simulink model "ENERGYMANAGEMENT0x2E"  (R2023b)
settings: Solver=VariableStepAuto  StartTime=0.0  StopTime=10  RelTol=1e-3  EnableMultiTasking=on
PreLoadFcn:
  |  SurfaceMountedPMSMFieldOrientedControlData
values from neighbouring files (symbols this model uses):
  F = 0.005    [SurfaceMountedPMSMFieldOrientedControlData.m]
  Fsw = 8000    [SurfaceMountedPMSMFieldOrientedControlData.m]
  Ts = 20e-6    (= 2e-05)    [SurfaceMountedPMSMFieldOrientedControlData.m]
undefined symbols (not defined in the file or in its folder): DiscIntNeverNeededParam, gcbh, Ion, Lithium, sps_rtmsupport
libraries: simulink x16, spsDiodeLib x6, spsSeriesRLCBranchLib x4, slpidlib x3, spsCurrentMeasurementLib x2, simulink_extras x2, spsMeanLib x2, spsSecondOrderFilterLib x2, spsIdealSwitchLib x2, spsPermanentMagnetSynchronousMachineLib x1, spsBatteryLib x1, spsMosfetLib x1
(part 1 of 2)
settings Model: SimulationMode=accelerator  Creator=The MathWorks, Inc.  LastModifiedBy=osman
settings SolverCC: AlgebraicLoopSolver=TrustRegion
settings DataIOCC: SaveOutput=off  SignalLogging=off  DSMLogging=off  SaveTime=off  ReturnWorkspaceOutputs=off
settings DebuggingCC: UnconnectedInputMsg=warning  UnconnectedOutputMsg=warning  UnconnectedLineMsg=warning
settings ModelReferenceCC: EnableRefExpFcnMdlSchedulingChecks=on
settings RTWCC: DLArmComputeVersion=19.05

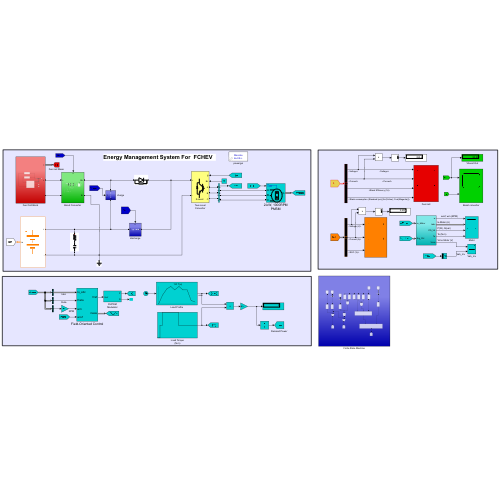
[thumbnail: Simulink's stored preview of the top-level diagram]
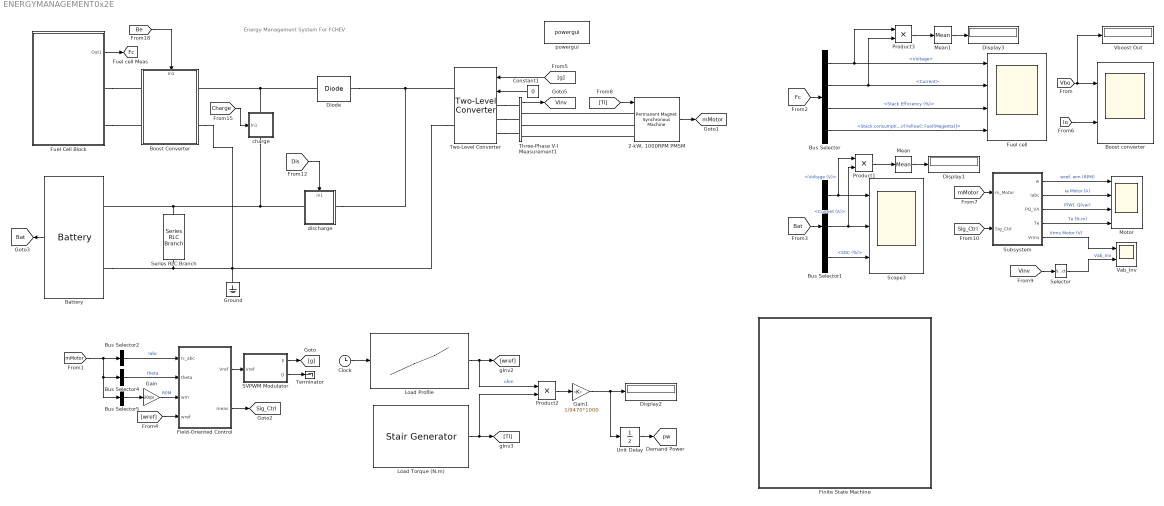
== system ENERGYMANAGEMENT0x2E ==
  note: Energy Management System For FCHEV
  "2-kW, 1000RPM PMSM" : spsPermanentMagnetSynchronousMachineLib/Permanent Magnet Synchronous Machine  NbPhases=3  FluxDistribution=Sinusoidal  RotorType=Round  MechanicalLoad=Torque Tm  PresetModel=No  ShowDetailedParameters=on  MeasurementBus=off  Resistance=0.01  Inductance=8.5e-3  dqInductances=[8.5e-3,8.5e-3]  La=0.002  MachineConstant=Flux linkage established by magnets (V.s)  Flux=0.175  VoltageCst=95.2245  TorqueCst=0.7875  Flat=120  Mechanical=[0.03 ,F 3]  PolePairs=2  InitialConditions=[0,0, 0,0]  InitialConditions5ph=[0 0 0 0 0 0]  RefAngle=90 degrees behind phase A axis (modified Park)  IterativeDiscreteModel=Trapezoidal robust  TsBlock=2e-5  TsPowergui=0
  Battery : spsBatteryLib/Battery  BatType=Lithium-Ion  ShowTempParam=off  ThermalPreset=no  ShowAgeParam=off  NomV=88  NomQ=11  SOC=75  Batt_Tr=30  PresetModel=on  MaxQ=11  MinV=66  FullV=102.4309  Dis_rate=4.7826  R=0.08  Normal_OP=9.9478  expZone="[95.074     0.540435]"  current=[6.5 13 32.5]  Units=Time  Tci=20  NomT=20  T2=-30  MaxQ2=4.8  FullV2=7.1  Normal_OP2=5.655  expZone2="[6.58           1]"  Rca=0.6  ti=2000  Dp=0  Neq0=0  Tsim=1e6  Ta1=25  Qeol=5.4*0.9  Reol=0.013333*1.2  Char_age=[2.3478, 3]  Dis_age=[2.3478, 10]  N1=1500  N2=10500  N3=1000  N4=1400  Ta2=45  N5=950
  Boost Converter : Subsystem
      settings: PortSchema="{\"entries\":[{\"content\":{\"sides\":[{\"content\":{\"connectorIds\":[\"LConn1\",\"LConn2\"]},\"type\":\"ConnectorPlacement.EquallySpacedRectSide\",\"uuid\":\"724820d7-5254-4590-9883-e42ece5a36b7\"},{\"content\":{\"connectorIds\":[\"RConn1\",\"RConn2\"],\"side\":\"RIGHT\"},\"type\":\"ConnectorPlacement.EquallySpacedRectSide\",\"uuid\":\"efd78358-38e4-437c-85ef-e8b0a8150418\"},{\"content\":{\"connectorIds\":[\"In1\"],\"side\":\"TOP\"},\"type\":\"ConnectorPlacement.EquallySpacedRectSide\",\"uuid\":\"51cbfe1b-7a5a-4465-8e4f-b2b0baad5ef4\"}]},\"type\":\"ConnectorPlacement.EquallySpacedConnector\",\"uuid\":\"bbc907d0-d787-42dc-8369-3440b3d38849\"}],\"packageUris\":[\"http://schema.mathworks.com/mf0/Connector/R2020b\"],\"version\":\"1.0\"}"
  Boost converter : Scope  NumInputPorts=2
  Bus Selector : BusSelector  OutputSignals=Voltage,Current,Stack Efficiency (%),Stack consumption (Standard lpm) [Air(Yellow); Fuel(Magenta)]
  Bus Selector1 : BusSelector  OutputSignals=Voltage (V),Current (A),SOC (%)
  Bus Selector2 : BusSelector  OutputSignals=Stator current is_a (A),Stator current is_b (A),Stator current is_c (A)  OutputAsBus=on
  Bus Selector4 : BusSelector  OutputSignals=Rotor angle thetam (rad)  OutputAsBus=on
  Bus Selector5 : BusSelector  OutputSignals=Rotor speed wm (rad/s)  OutputAsBus=on
  Clock : Clock
  Constant1 : Constant  Value=0
  Diode : spsDiodeLib/Diode  Ron=0.001  Lon=0  Vf=0.8  IC=0  UseSnubber=0  Rs=1e5  Cs=250e-9  Measurements=off
  Display1 : Display
  Display2 : Display
  Display3 : Display
  Field-Oriented Control : Subsystem  DialogController=POWERSYS.PowerSysDialog  LoadFcn=sps_rtmsupport('LoadFcn',gcbh);  StartFcn=sps_rtmsupport('StartFcn',gcbh);  StopFcn=sps_rtmsupport('StopFcn',gcbh);  mask(Field-Oriented Controller (FOC) of a PMSM drive){Kp_wreg=0.25, Ki_wreg=25, Limit_wreg=35, Kp_Ireg=0.2, Ki_Ireg=10, Limits_Ireg=2, p=3, Ts=2e-5}
      mask prompts: Kp_wreg "Proportional gain"; Ki_wreg "Integral gain"; Limit_wreg "Output (current) limit"; Kp_Ireg "Proportional gain"; Ki_Ireg "Integral gain"; Limits_Ireg "Output limit"; p "Number of pole pairs:"; Ts "Sample time (s)"
      settings: AttributesFormatString=\n  CopyFcn=sps_rtmsupport('CopyFcn',gcbh); powericon('psbloadfunction',gcbh,'gotofrom','UpdateGotoTag');  DeleteFcn=sps_rtmsupport('DeleteFcn',gcbh);  UndoDeleteFcn=sps_rtmsupport('UndoDeleteFcn',gcbh);  ModelCloseFcn=sps_rtmsupport('ModelCloseFcn',gcbh);  PreSaveFcn=sps_rtmsupport('PreSaveFcn',gcbh);  PostSaveFcn=sps_rtmsupport('PostSaveFcn',gcbh);  NameChangeFcn=sps_rtmsupport('NameChangeFcn',gcbh);  PreCopyFcn=sps_rtmsupport('PreCopyFcn',gcbh);  OpenFcn=sps_rtmsupport('OpenFcn',gcbh, [-1 2 -3 4 5 6 7 17 22 23]);  CloseFcn=sps_rtmsupport('CloseFcn',gcbh);  PreDeleteFcn=sps_rtmsupport('PreDeleteFcn',gcbh);
      mask Help: helpview(psbhelp);
      mask DialogControl Container11 Prompt: Control parameters
      mask DialogControl Container12 Prompt: Speed regulator
      mask DialogControl Container8 Prompt: Current regulators
  Finite State Machine : Subsystem
  Fuel Cell Block : Subsystem
  Fuel cell : Scope  NumInputPorts=4
  Gain : Gain  Gain=30/pi
  Gain1 : Gain  Gain=1/9470*1000
  Ground : spsGroundLib/Ground  LConnTagsString=a
  Load Profile : Lookup_n-D  NumberOfTableDimensions=1  BreakpointsForDimension1=[0 1 2 3 4 5 6 7 8 9 ]  BreakpointsForDimension2=[0 571.55 685.8 800.15 914.4 1028.8 1143.1 1257.4 1371.7 1486 1600.3 1714.6 1828.9 1943.2 2057.5 2171.8 2286.1 2400.5 2514.7 2629.1 2743.3 2857.7 2971.9 3086.3 3200.5 3314.9 3429.2]  Table=[0 500 850 1000 800 1000 800 800 200 100 ]  InternalRulePriority=Speed  RndMeth=Simplest
  Load Torque (N.m) : spsStairGeneratorLib/Stair Generator  t=[0 0.5 1 1.5 5 9]  e=[5 , 5 10 15 10 10 ]  Ts=Ts
  Mean : spsMeanLib/Mean  Freq=60  Vinit=0  Ts=2e-5
  Mean1 : spsMeanLib/Mean  Freq=60  Vinit=0  Ts=2e-5
  Motor : Scope  NumInputPorts=4
  Product1 : Product
  Product2 : Product
  Product3 : Product
  SVPWM Modulator : Subsystem  DialogController=POWERSYS.PowerSysDialog  LoadFcn=sps_rtmsupport('LoadFcn', gcbh);  StartFcn=sps_rtmsupport('StartFcn', gcbh);  StopFcn=sps_rtmsupport('StopFcn', gcbh);  mask(Unified PWM Modulator for a 2-level, 3-phase converter){PWMmethod=Space Vector PWM (SVPWM) with pulse averaging, Fsw=Fsw, Ts=Ts}
      mask prompts: PWMmethod "PWM method"; Fsw "Switching frequency (Hz):"; Ts "Sample time (s):"
      mask help:
      | Generate pulses for PWM-controlled two-level, three-phase power electronics converter with pulse averaging capability.
      |
      | The pulses generation can be perform using one of the following Pulse-Width Modulation (PWM) methods:
      | 1. Sinusoidal PWM (SPWM)
      | 2. Sinusoidal PWM (SPWM) with pulse averaging
      | 3. Space Vector PWM (SVPWM)
      | 4. Space Vector PWM (SVPWM) with pulse averaging
      | 5. 30 degrees discontinuous PWM
      |
      | When a PWM method with pulse averaging is selected, the output pulses are averaged over one sample time. (Pulses value will range from 0 to 1)
      mask init:
      | switch PWMmethod
      |     case 1 % SPWM
      |         ZeroOrderHold_Ts=-1;
      |         Pavg=0;
      |     case 2 % SPWM with pulse averaging
      |         ZeroOrderHold_Ts=-1;
      |         Pavg=1;
      |     case 3  % SVPWM
      |         ZeroOrderHold_Ts=-1;
      |         Pavg=0;
      |     case 4  % SVPWM with pulse averaging
      |         ZeroOrderHold_Ts=-1;
      |         Pavg=1;
      |     case 5  % 30 degrees discontinuous PWM
      |         ZeroOrderHold_Ts=1/Fsw/2;
      |         Pavg=0;
      | end
      settings: CopyFcn=sps_rtmsupport('CopyFcn', gcbh);  DeleteFcn=sps_rtmsupport('DeleteFcn', gcbh);  UndoDeleteFcn=sps_rtmsupport('UndoDeleteFcn', gcbh);  ModelCloseFcn=sps_rtmsupport('ModelCloseFcn', gcbh);  PreSaveFcn=sps_rtmsupport('PreSaveFcn', gcbh);  PostSaveFcn=sps_rtmsupport('PostSaveFcn', gcbh);  NameChangeFcn=sps_rtmsupport('NameChangeFcn', gcbh);  PreCopyFcn=sps_rtmsupport('PreCopyFcn', gcbh);  OpenFcn=sps_rtmsupport('OpenFcn', gcbh, [1]);  CloseFcn=sps_rtmsupport('CloseFcn', gcbh);  PreDeleteFcn=sps_rtmsupport('PreDeleteFcn', gcbh);
      mask TypeOptions PWMmethod: Sinusoidal PWM (SPWM) | Sinusoidal PWM (SPWM) wirh pulse averaging | Space Vector PWM (SVPWM) | Space Vector PWM (SVPWM) with pulse averaging | 30 degrees discontinuous PWM
  Scope3 : Scope  NumInputPorts=3
  Selector : Selector  InputPortWidth=3  IndexOptions=Index vector (dialog)  Indices=1  OutputSizes=1
  Series RLC Branch : spsSeriesRLCBranchLib/Series RLC Branch  LConnTagsString=__new0  RConnTagsString=__new0  BranchType=RC  Resistance=1  Inductance=1e-3  SetiL0=off  InitialCurrent=0  Capacitance=1e-4  Setx0=on  InitialVoltage=92  Measurements=None
  Subsystem : Subsystem
  Terminator : Terminator
  Three-Phase V-I Measurement1 : spsThreePhaseVIMeasurementLib/Three-Phase V-I Measurement  VoltageMeasurement=phase-to-phase  SetLabelV=off  LabelV=Vabc  Vpu=off  VpuLL=off  CurrentMeasurement=no  SetLabelI=off  LabelI=Iabc  Ipu=off  Pbase=100e6  Vbase=500e3  OutputType=Complex  PhasorSimulation=off  PSBequivalent=0
  Two-Level Converter : spsTwoLevelConverterLib/Two-Level Converter  ModelType=Switching function  Ron=1e-3  Rs=1e6  Cs=inf  Vforward=[0,0]  Ron_Diode=1e-3  Rs_Diode=1e6  Cs_Diode=inf  Vf_Diode=0  Rs_CurrentSource=inf  Ron_ACsource=1e-3
  Unit Delay : UnitDelay  SampleTime=2e-5  HasFrameUpgradeWarning=on
  Vab_Inv : Scope  NumInputPorts=2
  Vboost Out : Display
  charge : Subsystem
      settings: PortSchema="{\"entries\":[{\"content\":{\"sides\":[{\"content\":{\"connectorIds\":[\"LConn1\"]},\"type\":\"ConnectorPlacement.EquallySpacedRectSide\",\"uuid\":\"542812f3-0075-41f7-b004-faadc5b4cb6c\"},{\"content\":{\"connectorIds\":[\"RConn1\"],\"side\":\"RIGHT\"},\"type\":\"ConnectorPlacement.EquallySpacedRectSide\",\"uuid\":\"a1adf09c-e9ea-4226-86a1-520823d20346\"},{\"content\":{\"connectorIds\":[\"In1\"],\"side\":\"TOP\"},\"type\":\"ConnectorPlacement.EquallySpacedRectSide\",\"uuid\":\"e7c1831b-3d2b-475c-93da-3ac83c790107\"}]},\"type\":\"ConnectorPlacement.EquallySpacedConnector\",\"uuid\":\"19c42b2a-b3c4-4efa-a5c9-bfe092eb0a4e\"}],\"packageUris\":[\"http://schema.mathworks.com/mf0/Connector/R2020b\"],\"version\":\"1.0\"}"
  discharge : Subsystem
      settings: PortSchema="{\"entries\":[{\"content\":{\"sides\":[{\"content\":{\"connectorIds\":[\"LConn1\"]},\"type\":\"ConnectorPlacement.EquallySpacedRectSide\",\"uuid\":\"542812f3-0075-41f7-b004-faadc5b4cb6c\"},{\"content\":{\"connectorIds\":[\"RConn1\"],\"side\":\"RIGHT\"},\"type\":\"ConnectorPlacement.EquallySpacedRectSide\",\"uuid\":\"a1adf09c-e9ea-4226-86a1-520823d20346\"},{\"content\":{\"connectorIds\":[\"In1\"],\"side\":\"TOP\"},\"type\":\"ConnectorPlacement.EquallySpacedRectSide\",\"uuid\":\"e7c1831b-3d2b-475c-93da-3ac83c790107\"}]},\"type\":\"ConnectorPlacement.EquallySpacedConnector\",\"uuid\":\"19c42b2a-b3c4-4efa-a5c9-bfe092eb0a4e\"}],\"packageUris\":[\"http://schema.mathworks.com/mf0/Connector/R2020b\"],\"version\":\"1.0\"}"
  powergui : spspowerguiLib/powergui  Priority=1  SimulationMode=Discrete  SampleTime=Ts  frequency=60  Iterations=50  frequencyindice=0  Pbase=100e6  ErrMax=1e-4  UnitsV=kV  UnitsW=MW  buscounter=0  FunctionMessages=off  echomessages=off  EnableUseOfTLC=off  CurrentSourceSwitches=off  DisableSnubberDevices=off  DisableRonSwitches=off  DisableVfSwitches=off  DisplayEquations=off  AutomaticDiscreteSolvers=off  SolverType=Tustin/Backward Euler (TBE)  Interpol=off  ExternalGateDelay=off  methode=off  Ts=100  x0status=blocks  SPID=on  SwTol=0  HookPort=off  NonlinearTolerance=1e-4  nMaxIteration=100  ContinueOnMaxIteration=off  RestoreLinks=warning  ResistiveCurrentMeasurement=off  Frange=[0:2:500]  Ylog=off  Xlog=on  ShowGrid=off  save=off  variable=ZData  structure=Scope_Compare  ZoomFFT=off  StartTime=0.75  cycles=1  DisplayStyle=1  fundamental=100  FreqAxis=off  MaxFrequency=25000  frequencyindicesteady=1  RmsSteady=1  display=off
  tag scope: Bat=global, Fc=global, Sig_Ctrl=global, Vinv=global, mMotor=global, pw=global
  wires:
  Field-Oriented Control/1(Vref) -> SVPWM Modulator/1(Vref)
  Field-Oriented Control/2(meas) -> [Sig_Ctrl]
  [wref] -> Field-Oriented Control/4(wref)
  [mMotor] -> Bus Selector2/1, Bus Selector4/1, Bus Selector5/1
  Bus Selector2/1 -> Field-Oriented Control/1(Is_abc)  "Iabc"
  "2-kW, 1000RPM PMSM"/1 -> [mMotor]
  Constant1/1 -> Two-Level Converter/2
  Three-Phase V-I Measurement1/1 -> [Vinv]
  [g] -> Two-Level Converter/1
  Bus Selector5/1 -> Gain/1
  Gain/1 -> Field-Oriented Control/3(wm)  "RPM"
  Bus Selector4/1 -> Field-Oriented Control/2(theta)  "theta"
  SVPWM Modulator/1(P) -> [g]
  SVPWM Modulator/2(D) -> Terminator/1
  Battery/1 -> [Bat]
  Load Torque (N.m)/1 -> Product2/2, [Tl]
  Clock/1 -> Load Profile/1
  Load Profile/1 -> Product2/1, [wref]  "ohm"
  [Tl] -> "2-kW, 1000RPM PMSM"/1
  [Sig_Ctrl] -> Subsystem/2(Sig_Ctrl)
  Subsystem/3(PQ_VA) -> Motor/3  "P(W), Q(var)"
  [Vinv] -> Selector/1
  Subsystem/5(Vrms) -> Vab_Inv/1  "Vrms Motor (V)"
  Subsystem/4(Te) -> Motor/4  "Te (N.m)"
  [Bat] -> Bus Selector1/1
  Subsystem/2(Iabc) -> Motor/2  "Ia Motor (A)"
  [Vbo] -> Vboost Out/1, Boost converter/1
  Subsystem/1(w) -> Motor/1  "wref, wm (RPM)"
  Bus Selector/4 -> Fuel cell/4  "<Stack consumption (Standard lpm) [Air(Yellow); Fuel(Magenta)]>"
  Bus Selector/2 -> Product3/2, Fuel cell/2  "<Current>"
  [mMotor] -> Subsystem/1(m_Motor)
  [Fc] -> Bus Selector/1
  Bus Selector/3 -> Fuel cell/3  "<Stack Efficiency (%)>"
  Bus Selector/1 -> Product3/1, Fuel cell/1  "<Voltage>"
  [Io] -> Boost converter/2
  Selector/1 -> Vab_Inv/2  "Vab_Inv"
  Bus Selector1/1 -> Product1/1, Scope3/1  "<Voltage (V)>"
  Bus Selector1/2 -> Product1/2, Scope3/2  "<Current (A)>"
  Bus Selector1/3 -> Scope3/3  "<SOC (%)>"
  Fuel Cell Block/1(Out1) -> [Fc]
  Product2/1 -> Gain1/1
  Gain1/1 -> Unit Delay/1, Display2/1
  Unit Delay/1 -> [pw]
  [Dis] -> discharge/1(In1)
  [Charge] -> charge/1(In1)
  [Be] -> Boost Converter/1(In1)
  Product1/1 -> Mean/1
  Mean/1 -> Display1/1
  Mean1/1 -> Display3/1
  Product3/1 -> Mean1/1
  connections:
  "2-kW, 1000RPM PMSM"/LConn1 -- Three-Phase V-I Measurement1/RConn1
  Two-Level Converter/LConn3 -- Three-Phase V-I Measurement1/LConn3
  "2-kW, 1000RPM PMSM"/LConn2 -- Three-Phase V-I Measurement1/RConn2
  Two-Level Converter/LConn1 -- Three-Phase V-I Measurement1/LConn1
  Two-Level Converter/LConn2 -- Three-Phase V-I Measurement1/LConn2
  "2-kW, 1000RPM PMSM"/LConn3 -- Three-Phase V-I Measurement1/RConn3
  Fuel Cell Block/RConn2 -- Boost Converter/LConn2
  Fuel Cell Block/RConn1 -- Boost Converter/LConn1
  Two-Level Converter/RConn2 -- Series RLC Branch/RConn1 -- Battery/LConn2 -- Ground/LConn1 -- Boost Converter/RConn2
  discharge/LConn1 -- charge/RConn1 -- Series RLC Branch/LConn1 -- Battery/LConn1
  Diode/RConn1 -- discharge/RConn1 -- Two-Level Converter/RConn1
  Diode/LConn1 -- charge/LConn1 -- Boost Converter/RConn1

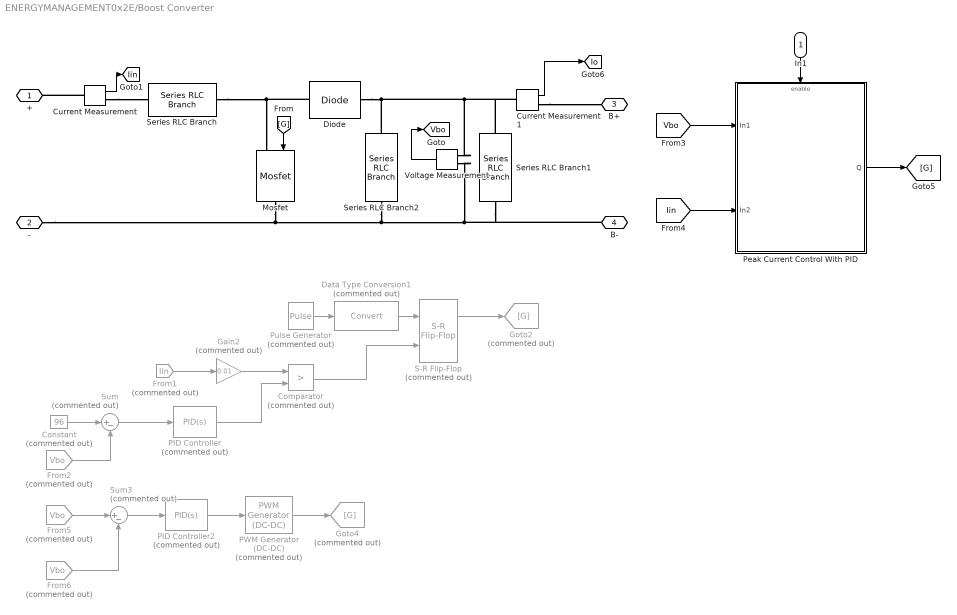
== system ENERGYMANAGEMENT0x2E/Boost Converter ==
  In1 : Inport
  Comparator : RelationalOperator  Commented=on  Operator=>  OutDataTypeStr=boolean  RndMeth=Simplest  InputSameDT=off
  Constant : Constant  Commented=on  Value=96
  Current Measurement : spsCurrentMeasurementLib/Current Measurement  PhasorSimulation=off  OutputType=Complex  PSBequivalent=0
  Current Measurement1 : spsCurrentMeasurementLib/Current Measurement  PhasorSimulation=off  OutputType=Complex  PSBequivalent=0
  Data Type Conversion1 : DataTypeConversion  Commented=on  SaturateOnIntegerOverflow=off  RndMeth=Floor
  Diode : spsDiodeLib/Diode  Ron=0.001  Lon=0  Vf=0  IC=0  UseSnubber=0  Rs=5e3  Cs=250e-9  Measurements=off
  From1 : From  Commented=on  GotoTag=Iin  TagVisibility=global
  From2 : From  Commented=on  GotoTag=Vbo  TagVisibility=global
  From5 : From  Commented=on  GotoTag=Vbo  TagVisibility=global
  From6 : From  Commented=on  GotoTag=Vbo  TagVisibility=global
  Gain2 : Gain  Commented=on  Gain=0.01
  Goto2 : Goto  Commented=on  GotoTag=G
  Goto4 : Goto  Commented=on  GotoTag=G
  Mosfet : spsMosfetLib/Mosfet  Ron=0.05  Lon=0  Rd=0.01  Vfd=0  IC=0  Rs=1e5  Cs=inf  Measurements=off
  PID Controller : slpidlib/PID Controller  Commented=on  Controller=PID  Form=Parallel  TimeDomain=Continuous-time  UseExternalTs=off  SampleTime=-1  IntegratorMethod=Forward Euler  FilterMethod=Forward Euler  ControllerParametersSource=internal  P=0.01  I=0.1  UseKiTs=off  D=0.001  N=100  UseFilter=on  TunerSelectOption=Transfer Function Based (PID Tuner App)  InitialConditionSource=internal  InitialConditionForIntegrator=0  InitialConditionForFilter=0  DifferentiatorICPrevScaledInput=0  ExternalReset=none  TrackingMode=off  Kt=1  LimitOutput=on  SatLimitsSource=internal  UpperSaturationLimit=0.80  LowerSaturationLimit=0  LinearizeAsGain=on  AntiWindupMode=none  Kb=1  LimitIntegrator=off  UpperIntegratorSaturationLimit=inf  LowerIntegratorSaturationLimit=-inf  POutMin=[]  POutMax=[]  IOutMin=[]  IOutMax=[]  DOutMin=[]  DOutMax=[]  NOutMin=[]  NOutMax=[]  SumOutMin=[]  SumOutMax=[]  SaturationOutMin=[]  SaturationOutMax=[]  PParamMin=[]  PParamMax=[]  IParamMin=[]  IParamMax=[]  DParamMin=[]  DParamMax=[]  NParamMin=[]  NParamMax=[]  KbParamMin=[]  KbParamMax=[]  KtParamMin=[]  KtParamMax=[]  KbOutMin=[]  KbOutMax=[]  KtOutMin=[]  KtOutMax=[]  IntegratorOutMin=[]  IntegratorOutMax=[]  FilterOutMin=[]  FilterOutMax=[]  SumI1OutMin=[]  SumI1OutMax=[]  SumI2OutMin=[]  SumI2OutMax=[]  SumI3OutMin=[]  SumI3OutMax=[]  SumI4OutMin=[]  SumI4OutMax=[]  SumDOutMin=[]  SumDOutMax=[]  DifferentiatorOutMin=[]  DifferentiatorOutMax=[]  FilterDiffOutCoefMin=[]  FilterDiffOutCoefMax=[]  ReciprocalOutMin=[]  ReciprocalOutMax=[]  SumDenOutMin=[]  SumDenOutMax=[]  SumNumOutMin=[]  SumNumOutMax=[]  DivideOutMin=[]  DivideOutMax=[]  UdiffTsProdOutMin=[]  UdiffTsProdOutMax=[]  NTsProdOutMin=[]  NTsProdOutMax=[]  UintegralTsProdOutMin=[]  UintegralTsProdOutMax=[]  UngainTsProdOutMin=[]  UngainTsProdOutMax=[]  ClampingZeroOutDataTypeStr=Inherit: Inherit via back propagation  ClampingZeroOutMin=[]  ClampingZeroOutMax=[]  FilterDenConstantOutDataTypeStr=Inherit: Inherit via back propagation  FilterDenConstantOutMin=[]  FilterDenConstantOutMax=[]  PCopyOutDataTypeStr=Inherit: Inherit via back propagation  PCopyOutMin=[]  PCopyOutMax=[]  NCopyOutDataTypeStr=Inherit: Inherit via back propagation  NCopyOutMin=[]  NCopyOutMax=[]  IntegratorContinuousStateAttributes=''  IntegratorStateMustResolveToSignalObject=off  IntegratorRTWStateStorageClass=Auto  FilterContinuousStateAttributes=''  FilterStateMustResolveToSignalObject=off  FilterRTWStateStorageClass=Auto  ParallelPVariant=InternalParameters  IdealPVariant=Disabled  IVariant=InternalParameters  DVariant=InternalParameters  IntegratorVariant=Continuous  SatVariant=Enabled  AWVariant=Passthrough  PCopyVariant=Disabled  TRVariant=Disabled  FdbkBlocksVariant=Forward  IdealPFdbkVariant=Disabled  SatFdbkVariant=Disabled  DerivativeFilterVariant=ContFilter  NVariant=InternalParameters  NCopyVariant=Disabled  FilterICVariant=InternalICsFilter  IntegratorICVariant=InternalICs  ExternalResetVariant=Disabled  TRSumVariant=Passthrough  SumFdbkVariant=Disabled  SumVariant=Sum_PID  TsampFilterVariant=InternalTs  TsampNgainVariant=Passthrough  TsampIntegralVariant=Disabled_SignalSpec  ExternalSaturationOutDataTypeStr=Inherit: Same as second input
  PID Controller2 : slpidlib/PID Controller  Commented=on  Controller=PID  Form=Parallel  TimeDomain=Continuous-time  UseExternalTs=off  SampleTime=-1  IntegratorMethod=Forward Euler  FilterMethod=Forward Euler  ControllerParametersSource=internal  P=0.01  I=0.1  UseKiTs=off  D=0.001  N=100  UseFilter=on  TunerSelectOption=Transfer Function Based (PID Tuner App)  InitialConditionSource=internal  InitialConditionForIntegrator=0  InitialConditionForFilter=0  DifferentiatorICPrevScaledInput=0  ExternalReset=none  TrackingMode=off  Kt=1  LimitOutput=on  SatLimitsSource=internal  UpperSaturationLimit=0.80  LowerSaturationLimit=0  LinearizeAsGain=on  AntiWindupMode=none  Kb=1  LimitIntegrator=off  UpperIntegratorSaturationLimit=inf  LowerIntegratorSaturationLimit=-inf  POutMin=[]  POutMax=[]  IOutMin=[]  IOutMax=[]  DOutMin=[]  DOutMax=[]  NOutMin=[]  NOutMax=[]  SumOutMin=[]  SumOutMax=[]  SaturationOutMin=[]  SaturationOutMax=[]  PParamMin=[]  PParamMax=[]  IParamMin=[]  IParamMax=[]  DParamMin=[]  DParamMax=[]  NParamMin=[]  NParamMax=[]  KbParamMin=[]  KbParamMax=[]  KtParamMin=[]  KtParamMax=[]  KbOutMin=[]  KbOutMax=[]  KtOutMin=[]  KtOutMax=[]  IntegratorOutMin=[]  IntegratorOutMax=[]  FilterOutMin=[]  FilterOutMax=[]  SumI1OutMin=[]  SumI1OutMax=[]  SumI2OutMin=[]  SumI2OutMax=[]  SumI3OutMin=[]  SumI3OutMax=[]  SumI4OutMin=[]  SumI4OutMax=[]  SumDOutMin=[]  SumDOutMax=[]  DifferentiatorOutMin=[]  DifferentiatorOutMax=[]  FilterDiffOutCoefMin=[]  FilterDiffOutCoefMax=[]  ReciprocalOutMin=[]  ReciprocalOutMax=[]  SumDenOutMin=[]  SumDenOutMax=[]  SumNumOutMin=[]  SumNumOutMax=[]  DivideOutMin=[]  DivideOutMax=[]  UdiffTsProdOutMin=[]  UdiffTsProdOutMax=[]  NTsProdOutMin=[]  NTsProdOutMax=[]  UintegralTsProdOutMin=[]  UintegralTsProdOutMax=[]  UngainTsProdOutMin=[]  UngainTsProdOutMax=[]  ClampingZeroOutDataTypeStr=Inherit: Inherit via back propagation  ClampingZeroOutMin=[]  ClampingZeroOutMax=[]  FilterDenConstantOutDataTypeStr=Inherit: Inherit via back propagation  FilterDenConstantOutMin=[]  FilterDenConstantOutMax=[]  PCopyOutDataTypeStr=Inherit: Inherit via back propagation  PCopyOutMin=[]  PCopyOutMax=[]  NCopyOutDataTypeStr=Inherit: Inherit via back propagation  NCopyOutMin=[]  NCopyOutMax=[]  IntegratorContinuousStateAttributes=''  IntegratorStateMustResolveToSignalObject=off  IntegratorRTWStateStorageClass=Auto  FilterContinuousStateAttributes=''  FilterStateMustResolveToSignalObject=off  FilterRTWStateStorageClass=Auto  ParallelPVariant=InternalParameters  IdealPVariant=Disabled  IVariant=InternalParameters  DVariant=InternalParameters  IntegratorVariant=Continuous  SatVariant=Enabled  AWVariant=Passthrough  PCopyVariant=Disabled  TRVariant=Disabled  FdbkBlocksVariant=Forward  IdealPFdbkVariant=Disabled  SatFdbkVariant=Disabled  DerivativeFilterVariant=ContFilter  NVariant=InternalParameters  NCopyVariant=Disabled  FilterICVariant=InternalICsFilter  IntegratorICVariant=InternalICs  ExternalResetVariant=Disabled  TRSumVariant=Passthrough  SumFdbkVariant=Disabled  SumVariant=Sum_PID  TsampFilterVariant=InternalTs  TsampNgainVariant=Passthrough  TsampIntegralVariant=Disabled_SignalSpec  ExternalSaturationOutDataTypeStr=Inherit: Same as second input
  PWM Generator (DC-DC) : spsPWMGeneratorDCDCLib/PWM Generator (DC-DC)  Commented=on  Fsw=500e3  Ts=0
  Peak Current Control With PID : Subsystem
  Pulse Generator : DiscretePulseGenerator  Commented=on  PulseType=Time based  Period=1e-5  PulseWidth=0.1
  S-R Flip-Flop : simulink_extras/Flip Flops/S-R Flip-Flop  Commented=on  initial_condition=0
  Series RLC Branch : spsSeriesRLCBranchLib/Series RLC Branch  LConnTagsString=__new0  RConnTagsString=__new0  BranchType=L  Resistance=0.01  Inductance=1e-3  SetiL0=off  InitialCurrent=0  Capacitance=1e-6  Setx0=off  InitialVoltage=0  Measurements=None
  Series RLC Branch1 : spsSeriesRLCBranchLib/Series RLC Branch  LConnTagsString=__new0  RConnTagsString=__new0  BranchType=R  Resistance=1e3  Inductance=20e-3  SetiL0=off  InitialCurrent=0  Capacitance=2e-1  Setx0=off  InitialVoltage=96  Measurements=None
  Series RLC Branch2 : spsSeriesRLCBranchLib/Series RLC Branch  LConnTagsString=__new0  RConnTagsString=__new0  BranchType=C  Resistance=0.01  Inductance=20e-3  SetiL0=off  InitialCurrent=0  Capacitance=80e-3  Setx0=off  InitialVoltage=96  Measurements=None
  Sum : Sum  Commented=on  Inputs=|+-
  Sum3 : Sum  Commented=on  Inputs=|+-
  Voltage Measurement : spsVoltageMeasurementLib/Voltage Measurement  PhasorSimulation=off  OutputType=Complex  PSBequivalent=0
  + : PMIOPort  Side=Left
  - : PMIOPort  Port=2  Side=Left
  B+ : PMIOPort  Port=3  Side=Right
  B- : PMIOPort  Port=4  Side=Right
  tag scope: Iin=global, Io=global, Vbo=global
  wires:
  Voltage Measurement/1 -> [Vbo]
  Current Measurement/1 -> [Iin]
  [G] -> Mosfet/1
  From2/1 -> Sum/2
  Sum/1 -> PID Controller/1
  Constant/1 -> Sum/1
  S-R Flip-Flop/1 -> Goto2/1
  Pulse Generator/1 -> Data Type Conversion1/1
  Data Type Conversion1/1 -> S-R Flip-Flop/1
  Comparator/1 -> S-R Flip-Flop/2
  PWM Generator (DC-DC)/1 -> Goto4/1
  PID Controller/1 -> Comparator/2
  Gain2/1 -> Comparator/1
  From1/1 -> Gain2/1
  Current Measurement1/1 -> [Io]
  PID Controller2/1 -> PWM Generator (DC-DC)/1
  Sum3/1 -> PID Controller2/1
  From5/1 -> Sum3/1
  From6/1 -> Sum3/2
  [Vbo] -> Peak Current Control With PID/1(In1)
  [Iin] -> Peak Current Control With PID/2(In2)
  Peak Current Control With PID/1(Q) -> [G]
  In1/1 -> Peak Current Control With PID/Enable
  connections:
  Diode/LConn1 -- Series RLC Branch/RConn1 -- Mosfet/LConn1
  Mosfet/RConn1 -- -/RConn1 -- Series RLC Branch2/RConn1 -- Voltage Measurement/LConn2 -- Series RLC Branch1/RConn1 -- B-/RConn1
  Current Measurement/LConn1 -- +/RConn1
  Diode/RConn1 -- Current Measurement1/LConn1 -- Series RLC Branch1/LConn1 -- Voltage Measurement/LConn1 -- Series RLC Branch2/LConn1
  Current Measurement/RConn1 -- Series RLC Branch/LConn1
  Current Measurement1/RConn1 -- B+/RConn1

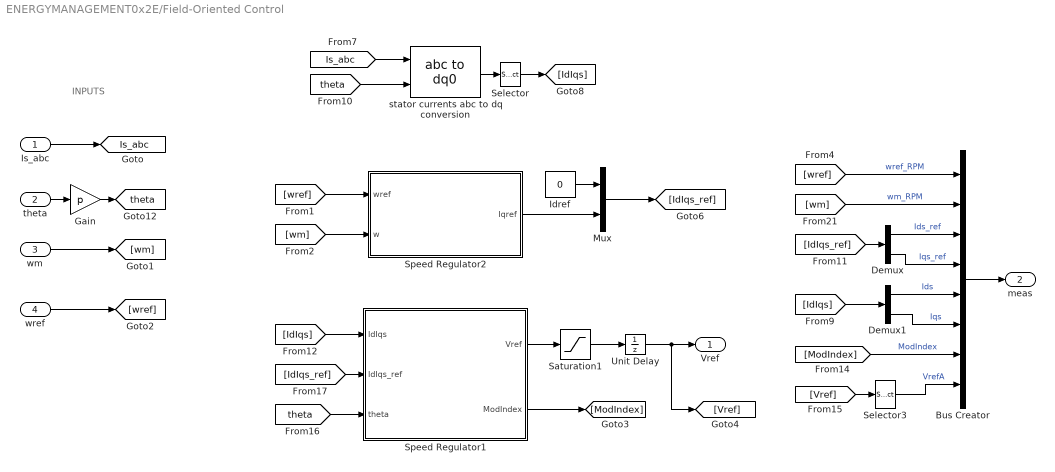
== system ENERGYMANAGEMENT0x2E/Field-Oriented Control ==
  note: INPUTS
  Is_abc : Inport  PortDimensions=3
  theta : Inport  Port=2  PortDimensions=1
  wm : Inport  Port=3  PortDimensions=1
  wref : Inport  Port=4  PortDimensions=1
  Bus Creator : BusCreator  Inputs=8
  Demux : Demux  Outputs=2
  Demux1 : Demux  Outputs=2
  Gain : Gain  Gain=p
  Idref : Constant  Value=0  SampleTime=Ts
  Mux : Mux  Inputs=2
  Saturation1 : Saturate  UpperLimit=2/sqrt(3)  LowerLimit=-2/sqrt(3)
  Selector : Selector  InputPortWidth=3  IndexOptions=Index vector (dialog)  Indices=[1 2]  OutputSizes=1
  Selector3 : Selector  InputPortWidth=3  IndexOptions=Index vector (dialog)  Indices=1  OutputSizes=1
  Speed Regulator1 : Subsystem  DialogController=POWERSYS.PowerSysDialog  mask(Current Regulators){Kp=Kp_Ireg, Ki=Ki_Ireg, Limits=Limits_Ireg, Init=0, Ts=Ts}
      mask prompts: Kp "Proportional gain (Kp):"; Ki "Integral gain (Ki):"; Limits "Output limits"; Init "Output initial value:"; Ts "Sample time:"
      mask help: This block implements two current regulators (Id & Iq) using anti-windup PI controllers.
      mask Display: disp('Current\nRegulators');
  Speed Regulator2 : Subsystem  DialogController=POWERSYS.PowerSysDialog  mask(Speed Regulator){Kp=Kp_wreg, Ki=Ki_wreg, Limit_wreg=Limit_wreg, Init=0, Ts=Ts}
      mask prompts: Kp "Proportional gain (Kp):"; Ki "Integral gain (Ki):"; Limit_wreg "Output limits"; Init "Output initial value:"; Ts "Sample time:"
      mask help: This block implements a speed regulator using an ant-windup PI controller.
      mask Display: disp('Speed\nRegulator');
  Unit Delay : UnitDelay  SampleTime=-1  HasFrameUpgradeWarning=on
  stator currents abc to dq conversion : spsabctodq0Lib/abc to dq0  Alignment=90 degrees behind phase A axis
  Vref : Outport  PortDimensions=3
  meas : Outport  Port=2
  tag scope: Is_abc=global, theta=global
  wires:
  Gain/1 -> [theta]
  Selector3/1 -> Bus Creator/8  "VrefA"
  [ModIndex] -> Bus Creator/7  "ModIndex"
  Mux/1 -> [IdIqs_ref]
  [IdIqs_ref] -> Speed Regulator1/2(IdIqs_ref)
  Idref/1 -> Mux/1
  Speed Regulator2/1(Iqref) -> Mux/2
  wref/1 -> [wref]
  theta/1 -> Gain/1
  Saturation1/1 -> Unit Delay/1
  [Vref] -> Selector3/1
  Speed Regulator1/2(ModIndex) -> [ModIndex]
  [IdIqs] -> Demux1/1
  Demux1/2 -> Bus Creator/6  "Iqs"
  Demux1/1 -> Bus Creator/5  "Ids"
  [IdIqs_ref] -> Demux/1
  Demux/2 -> Bus Creator/4  "Iqs_ref"
  Demux/1 -> Bus Creator/3  "Ids_ref"
  [wm] -> Bus Creator/2  "wm_RPM"
  [wref] -> Bus Creator/1  "wref_RPM"
  [IdIqs] -> Speed Regulator1/1(IdIqs)
  [theta] -> Speed Regulator1/3(theta)
  Is_abc/1 -> [Is_abc]
  Speed Regulator1/1(Vref) -> Saturation1/1
  stator currents abc to dq conversion/1 -> Selector/1
  [theta] -> stator currents abc to dq conversion/2
  [wm] -> Speed Regulator2/2(w)
  [wref] -> Speed Regulator2/1(wref)
  [Is_abc] -> stator currents abc to dq conversion/1
  Selector/1 -> [IdIqs]
  Unit Delay/1 -> [Vref], Vref/1
  Bus Creator/1 -> meas/1
  wm/1 -> [wm]

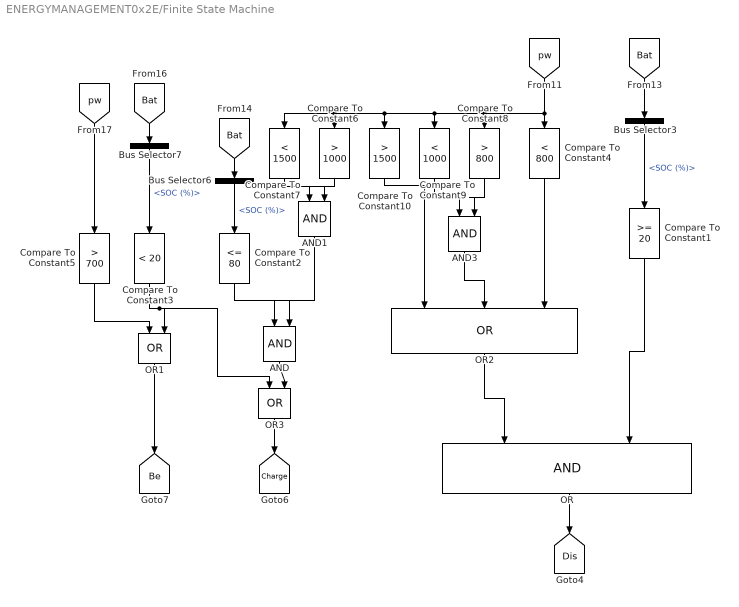
== system ENERGYMANAGEMENT0x2E/Finite State Machine ==
  AND : Logic  IconShape=distinctive  AllPortsSameDT=off  OutDataTypeStr=boolean
  AND1 : Logic  IconShape=distinctive  AllPortsSameDT=off  OutDataTypeStr=boolean
  AND3 : Logic  IconShape=distinctive  AllPortsSameDT=off  OutDataTypeStr=boolean
  Bus Selector3 : BusSelector  OutputSignals=SOC (%)
  Bus Selector6 : BusSelector  OutputSignals=SOC (%)
  Bus Selector7 : BusSelector  OutputSignals=SOC (%)
  Compare To Constant1 : simulink/Logic and Bit Operations/Compare To Constant  relop=>=  const=20  OutDataTypeStr=boolean
  Compare To Constant10 : simulink/Logic and Bit Operations/Compare To Constant  relop=>  const=1500  OutDataTypeStr=boolean
  Compare To Constant2 : simulink/Logic and Bit Operations/Compare To Constant  relop=<=  const=80  OutDataTypeStr=boolean
  Compare To Constant3 : simulink/Logic and Bit Operations/Compare To Constant  relop=<  const=20  OutDataTypeStr=boolean
  Compare To Constant4 : simulink/Logic and Bit Operations/Compare To Constant  relop=<  const=800  OutDataTypeStr=boolean
  Compare To Constant5 : simulink/Logic and Bit Operations/Compare To Constant  relop=>  const=700  OutDataTypeStr=boolean
  Compare To Constant6 : simulink/Logic and Bit Operations/Compare To Constant  relop=>  const=1000  OutDataTypeStr=boolean
  Compare To Constant7 : simulink/Logic and Bit Operations/Compare To Constant  relop=<  const=1500  OutDataTypeStr=boolean
  Compare To Constant8 : simulink/Logic and Bit Operations/Compare To Constant  relop=>  const=800  OutDataTypeStr=boolean
  Compare To Constant9 : simulink/Logic and Bit Operations/Compare To Constant  relop=<  const=1000  OutDataTypeStr=boolean
  OR : Logic  AllPortsSameDT=off  OutDataTypeStr=boolean
  OR1 : Logic  Operator=OR  IconShape=distinctive  AllPortsSameDT=off  OutDataTypeStr=boolean
  OR2 : Logic  Operator=OR  Inputs=3  AllPortsSameDT=off  OutDataTypeStr=boolean
  OR3 : Logic  Operator=OR  IconShape=distinctive  AllPortsSameDT=off  OutDataTypeStr=boolean
  tag scope: Be=global, Charge=global, Dis=global
  wires:
  [pw] -> Compare To Constant6/1, Compare To Constant7/1, Compare To Constant10/1, Compare To Constant9/1, Compare To Constant8/1, Compare To Constant4/1
  Bus Selector7/1 -> Compare To Constant3/1  "<SOC (%)>"
  [pw] -> Compare To Constant5/1
  Compare To Constant2/1 -> AND/2
  [Bat] -> Bus Selector3/1
  OR1/1 -> [Be]
  OR/1 -> [Dis]
  [Bat] -> Bus Selector6/1
  [Bat] -> Bus Selector7/1
  Bus Selector6/1 -> Compare To Constant2/1  "<SOC (%)>"
  AND1/1 -> AND/1
  OR3/1 -> [Charge]
  Bus Selector3/1 -> Compare To Constant1/1  "<SOC (%)>"
  Compare To Constant7/1 -> AND1/2
  Compare To Constant6/1 -> AND1/1
  Compare To Constant10/1 -> OR2/1
  AND3/1 -> OR2/2
  Compare To Constant4/1 -> OR2/3
  Compare To Constant9/1 -> AND3/1
  Compare To Constant8/1 -> AND3/2
  OR2/1 -> OR/1
  Compare To Constant1/1 -> OR/2
  Compare To Constant3/1 -> OR3/1, OR1/2
  Compare To Constant5/1 -> OR1/1
  AND/1 -> OR3/2

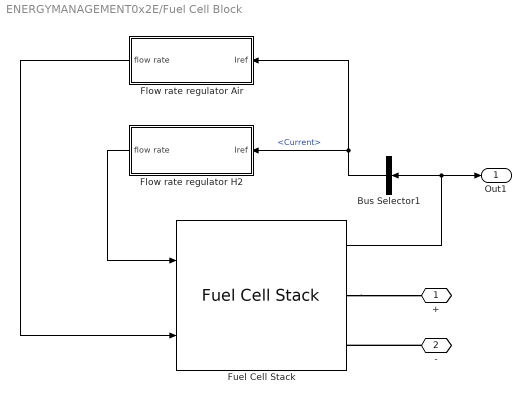
== system ENERGYMANAGEMENT0x2E/Fuel Cell Block ==
  Bus Selector1 : BusSelector  OutputSignals=Current
  Flow rate regulator Air : Subsystem
  Flow rate regulator H2 : Subsystem
  Fuel Cell Stack : spsFuelCellStackLib/Fuel Cell Stack  PresetModel=No (User-Defined)  FcType=Proton Exchange Membrane (PEM)  Detailed=Detailed  Eoc=[48,45]  NomVI=[42,36]  EndVI=[85,24]  Nc=52  n=55  TOp=65  AirFr=100  SuppPress=[1.5,1]  Comp=[99.95,21,1]  SignX=off  SignY=off  FlowRateH2=on  FlowRateAir=on  SystemTemp=off  SystemPH2=off  SystemPAir=off  FCDyn=on  FC_tau=2  Peak_O2=60  V_Under=2
      settings: LibrarySourceBlock=electricdrivelib/Extra Sources/Fuel Cell Stack
  + : PMIOPort  Side=Right
  - : PMIOPort  Port=2  Side=Right
  Out1 : Outport
  wires:
  Bus Selector1/1 -> Flow rate regulator Air/1(Iref), Flow rate regulator H2/1(Iref)  "<Current>"
  Flow rate regulator Air/1(flow rate) -> Fuel Cell Stack/2
  Fuel Cell Stack/1 -> Out1/1, Bus Selector1/1
  Flow rate regulator H2/1(flow rate) -> Fuel Cell Stack/1
  connections:
  -/RConn1 -- Fuel Cell Stack/RConn2
  Fuel Cell Stack/RConn1 -- +/RConn1

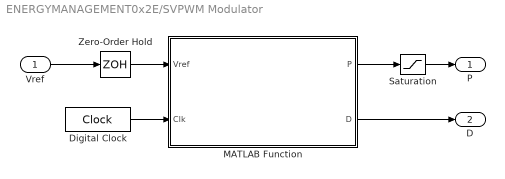
== system ENERGYMANAGEMENT0x2E/SVPWM Modulator ==
  Vref : Inport  PortDimensions=3  SampleTime=Ts
  Digital Clock : DigitalClock  SampleTime=Ts
  MATLAB Function : MATLAB Function  TreatAsAtomicUnit=on
  Saturation : Saturate  UpperLimit=1  LowerLimit=0
  Zero-Order Hold : ZeroOrderHold  SampleTime=ZeroOrderHold_Ts
  P : Outport  PortDimensions=6  SampleTime=Ts  VectorParamsAs1DForOutWhenUnconnected=off
  D : Outport  Port=2  PortDimensions=3  SampleTime=Ts  VectorParamsAs1DForOutWhenUnconnected=off
  wires:
  MATLAB Function/2(D) -> D/1
  MATLAB Function/1(P) -> Saturation/1
  Vref/1 -> Zero-Order Hold/1
  Saturation/1 -> P/1
  Digital Clock/1 -> MATLAB Function/2(Clk)
  Zero-Order Hold/1 -> MATLAB Function/1(Vref)

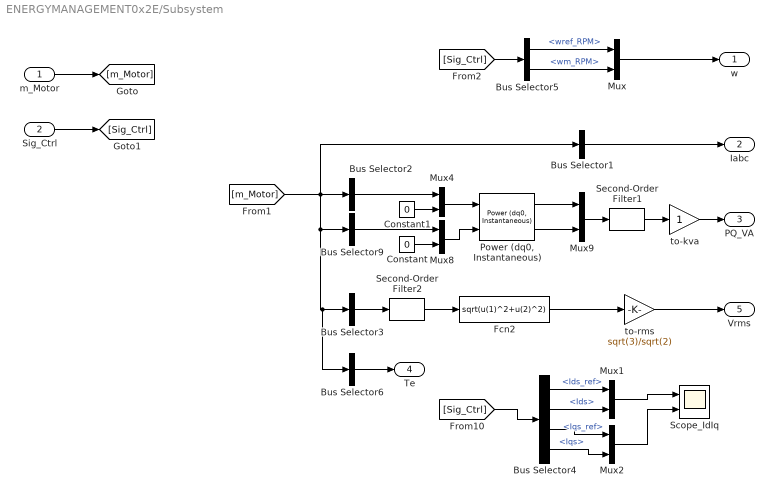
== system ENERGYMANAGEMENT0x2E/Subsystem ==
  m_Motor : Inport
  Sig_Ctrl : Inport  Port=2
  Bus Selector1 : BusSelector  OutputSignals=Stator current is_a (A),Stator current is_b (A),Stator current is_c (A)  OutputAsBus=on
  Bus Selector2 : BusSelector  OutputSignals=Stator voltage Vs_d (V),Stator voltage Vs_q (V)  OutputAsBus=on
  Bus Selector3 : BusSelector  OutputSignals=Stator voltage Vs_d (V),Stator voltage Vs_q (V)  OutputAsBus=on
  Bus Selector4 : BusSelector  OutputSignals=Ids_ref,Ids,Iqs_ref,Iqs
  Bus Selector5 : BusSelector  OutputSignals=wref_RPM,wm_RPM
  Bus Selector6 : BusSelector  OutputSignals=Electromagnetic torque Te (N*m)  OutputAsBus=on
  Bus Selector9 : BusSelector  OutputSignals=Stator current is_d (A),Stator current is_q (A)  OutputAsBus=on
  Constant : Constant  Value=0
  Constant1 : Constant  Value=0
  Fcn2 : Fcn  Expr=sqrt(u(1)^2+u(2)^2)
  Mux{,1..2,9} (4 alike) : Mux  Inputs=2
  Mux4 : Mux  Inputs=[2, 1]
  Mux8 : Mux  Inputs=[2, 1]
  "Power (dq0, Instantaneous)" : spsPowerdq0InstantaneousLib/Power (dq0, Instantaneous)
  Scope_IdIq : Scope  NumInputPorts=2
  Second-Order Filter1 : spsSecondOrderFilterLib/Second-Order Filter  FilterType=Lowpass  Fo=80  Zeta=1  Ts=Ts  Initialize=off  Vac_Init="[0,  0,  60]"  Vdc_Init=0  PlotResponse=off  FreqRange=[0, 500, 1]
  Second-Order Filter2 : spsSecondOrderFilterLib/Second-Order Filter  FilterType=Lowpass  Fo=120  Zeta=1  Ts=Ts  Initialize=off  Vac_Init="[0,  0,  60]"  Vdc_Init=0  PlotResponse=off  FreqRange=[0, 500, 1]
  to-kva : Gain
  to-rms : Gain  Gain=sqrt(3)/sqrt(2)
  w : Outport
  Iabc : Outport  Port=2
  PQ_VA : Outport  Port=3
  Te : Outport  Port=4
  Vrms : Outport  Port=5
  wires:
  Bus Selector6/1 -> Te/1
  Mux2/1 -> Scope_IdIq/2
  Mux1/1 -> Scope_IdIq/1
  Bus Selector4/4 -> Mux2/2  "<Iqs>"
  Bus Selector4/3 -> Mux2/1  "<Iqs_ref>"
  Bus Selector4/2 -> Mux1/2  "<Ids>"
  Bus Selector4/1 -> Mux1/1  "<Ids_ref>"
  Bus Selector1/1 -> Iabc/1
  Bus Selector5/2 -> Mux/2  "<wm_RPM>"
  Bus Selector5/1 -> Mux/1  "<wref_RPM>"
  [Sig_Ctrl] -> Bus Selector5/1
  [Sig_Ctrl] -> Bus Selector4/1
  Mux/1 -> w/1
  Mux8/1 -> "Power (dq0, Instantaneous)"/2
  Second-Order Filter2/1 -> Fcn2/1
  Fcn2/1 -> to-rms/1
  to-kva/1 -> PQ_VA/1
  to-rms/1 -> Vrms/1
  Mux9/1 -> Second-Order Filter1/1
  "Power (dq0, Instantaneous)"/1 -> Mux9/1
  Bus Selector2/1 -> Mux4/1
  "Power (dq0, Instantaneous)"/2 -> Mux9/2
  Constant/1 -> Mux8/2
  Bus Selector9/1 -> Mux8/1
  Constant1/1 -> Mux4/2
  Bus Selector3/1 -> Second-Order Filter2/1
  Mux4/1 -> "Power (dq0, Instantaneous)"/1
  [m_Motor] -> Bus Selector3/1, Bus Selector6/1, Bus Selector9/1, Bus Selector1/1, Bus Selector2/1
  m_Motor/1 -> [m_Motor]
  Sig_Ctrl/1 -> [Sig_Ctrl]
  Second-Order Filter1/1 -> to-kva/1

== system ENERGYMANAGEMENT0x2E/charge ==
  In1 : Inport
  Diode1 : spsDiodeLib/Diode  Ron=0.001  Lon=0  Vf=0.8  IC=0  UseSnubber=0  Rs=500  Cs=250e-9  Measurements=off
  Diode2 : spsDiodeLib/Diode  Ron=0.001  Lon=0  Vf=0.8  IC=0  UseSnubber=0  Rs=1e5  Cs=250e-9  Measurements=off
  Ideal Switch : spsIdealSwitchLib/Ideal Switch  Ron=0.001  Lon=0  IC=0  Rs=1e5  Cs=inf  Measurements=off
  1 : PMIOPort  Side=Left
  2 : PMIOPort  Port=2  Side=Right
  wires:
  In1/1 -> Ideal Switch/1
  connections:
  Ideal Switch/LConn1 -- Diode1/RConn1
  1/RConn1 -- Diode1/LConn1
  Diode2/RConn1 -- 2/RConn1
  Diode2/LConn1 -- Ideal Switch/RConn1

== system ENERGYMANAGEMENT0x2E/discharge ==
  In1 : Inport
  Diode1 : spsDiodeLib/Diode  Ron=0.001  Lon=0  Vf=0.8  IC=0  UseSnubber=0  Rs=500  Cs=250e-9  Measurements=off
  Diode2 : spsDiodeLib/Diode  Ron=0.001  Lon=0  Vf=0.8  IC=0  UseSnubber=0  Rs=1e5  Cs=250e-9  Measurements=off
  Ideal Switch : spsIdealSwitchLib/Ideal Switch  Ron=0.001  Lon=0  IC=0  Rs=1e5  Cs=inf  Measurements=off
  1 : PMIOPort  Side=Left
  2 : PMIOPort  Port=2  Side=Right
  wires:
  In1/1 -> Ideal Switch/1
  connections:
  1/RConn1 -- Diode1/LConn1
  Ideal Switch/LConn1 -- Diode1/RConn1
  Diode2/LConn1 -- Ideal Switch/RConn1
  2/RConn1 -- Diode2/RConn1

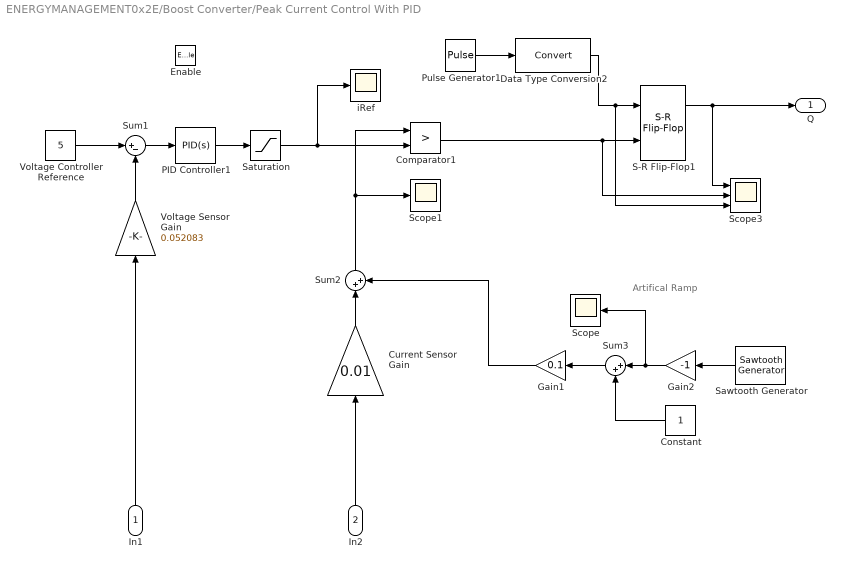
== system ENERGYMANAGEMENT0x2E/Boost Converter/Peak Current Control With PID ==
  note: Artifical Ramp
  In1 : Inport
  In2 : Inport  Port=2
  Enable : EnablePort
  Comparator1 : RelationalOperator  Operator=>  OutDataTypeStr=boolean  RndMeth=Simplest  InputSameDT=off
  Constant : Constant
  Current Sensor Gain : Gain  Gain=0.01
  Data Type Conversion2 : DataTypeConversion  SaturateOnIntegerOverflow=off  RndMeth=Floor
  Gain1 : Gain  Gain=0.1
  Gain2 : Gain  Gain=-1
  PID Controller1 : slpidlib/PID Controller  Controller=PID  Form=Parallel  TimeDomain=Continuous-time  UseExternalTs=off  SampleTime=-1  IntegratorMethod=Forward Euler  FilterMethod=Forward Euler  ControllerParametersSource=internal  P=0.3  I=0.6  UseKiTs=off  D=0.01  N=100  UseFilter=on  TunerSelectOption=Transfer Function Based (PID Tuner App)  InitialConditionSource=internal  InitialConditionForIntegrator=0  InitialConditionForFilter=0  DifferentiatorICPrevScaledInput=0  ExternalReset=none  TrackingMode=off  Kt=1  LimitOutput=off  SatLimitsSource=internal  UpperSaturationLimit=0.75  LowerSaturationLimit=0  LinearizeAsGain=on  AntiWindupMode=none  Kb=1  LimitIntegrator=off  UpperIntegratorSaturationLimit=inf  LowerIntegratorSaturationLimit=-inf  POutMin=[]  POutMax=[]  IOutMin=[]  IOutMax=[]  DOutMin=[]  DOutMax=[]  NOutMin=[]  NOutMax=[]  SumOutMin=[]  SumOutMax=[]  SaturationOutMin=[]  SaturationOutMax=[]  PParamMin=[]  PParamMax=[]  IParamMin=[]  IParamMax=[]  DParamMin=[]  DParamMax=[]  NParamMin=[]  NParamMax=[]  KbParamMin=[]  KbParamMax=[]  KtParamMin=[]  KtParamMax=[]  KbOutMin=[]  KbOutMax=[]  KtOutMin=[]  KtOutMax=[]  IntegratorOutMin=[]  IntegratorOutMax=[]  FilterOutMin=[]  FilterOutMax=[]  SumI1OutMin=[]  SumI1OutMax=[]  SumI2OutMin=[]  SumI2OutMax=[]  SumI3OutMin=[]  SumI3OutMax=[]  SumI4OutMin=[]  SumI4OutMax=[]  SumDOutMin=[]  SumDOutMax=[]  DifferentiatorOutMin=[]  DifferentiatorOutMax=[]  FilterDiffOutCoefMin=[]  FilterDiffOutCoefMax=[]  ReciprocalOutMin=[]  ReciprocalOutMax=[]  SumDenOutMin=[]  SumDenOutMax=[]  SumNumOutMin=[]  SumNumOutMax=[]  DivideOutMin=[]  DivideOutMax=[]  UdiffTsProdOutMin=[]  UdiffTsProdOutMax=[]  NTsProdOutMin=[]  NTsProdOutMax=[]  UintegralTsProdOutMin=[]  UintegralTsProdOutMax=[]  UngainTsProdOutMin=[]  UngainTsProdOutMax=[]  ClampingZeroOutDataTypeStr=Inherit: Inherit via back propagation  ClampingZeroOutMin=[]  ClampingZeroOutMax=[]  FilterDenConstantOutDataTypeStr=Inherit: Inherit via back propagation  FilterDenConstantOutMin=[]  FilterDenConstantOutMax=[]  PCopyOutDataTypeStr=Inherit: Inherit via back propagation  PCopyOutMin=[]  PCopyOutMax=[]  NCopyOutDataTypeStr=Inherit: Inherit via back propagation  NCopyOutMin=[]  NCopyOutMax=[]  IntegratorContinuousStateAttributes=''  IntegratorStateMustResolveToSignalObject=off  IntegratorRTWStateStorageClass=Auto  FilterContinuousStateAttributes=''  FilterStateMustResolveToSignalObject=off  FilterRTWStateStorageClass=Auto  ParallelPVariant=InternalParameters  IdealPVariant=Disabled  IVariant=InternalParameters  DVariant=InternalParameters  IntegratorVariant=Continuous  SatVariant=Disabled  AWVariant=Passthrough  PCopyVariant=Disabled  TRVariant=Disabled  FdbkBlocksVariant=Forward  IdealPFdbkVariant=Disabled  SatFdbkVariant=Disabled  DerivativeFilterVariant=ContFilter  NVariant=InternalParameters  NCopyVariant=Disabled  FilterICVariant=InternalICsFilter  IntegratorICVariant=InternalICs  ExternalResetVariant=Disabled  TRSumVariant=Passthrough  SumFdbkVariant=Disabled  SumVariant=Sum_PID  TsampFilterVariant=InternalTs  TsampNgainVariant=Passthrough  TsampIntegralVariant=Disabled_SignalSpec  ExternalSaturationOutDataTypeStr=Inherit: Same as second input
  Pulse Generator1 : DiscretePulseGenerator  PulseType=Time based  Period=1e-5  PulseWidth=0.001
  S-R Flip-Flop1 : simulink_extras/Flip Flops/S-R Flip-Flop  initial_condition=0
  Saturation : Saturate  UpperLimit=0.6  LowerLimit=0
  Sawtooth Generator : spsSawtoothGeneratorLib/Sawtooth Generator  Freq=1e3  Phase=0  Ts=0
  Scope : Scope
  Scope1 : Scope
  Scope3 : Scope  NumInputPorts=3
  Sum1 : Sum  Inputs=|+-
  Sum2 : Sum  Inputs=|++
  Sum3 : Sum  Inputs=|++
  Voltage Controller Reference : Constant  Value=5
  Voltage Sensor Gain : Gain  Gain=0.052083
  iRef : Scope
  Q : Outport
  wires:
  Sum2/1 -> Scope1/1, Comparator1/1
  S-R Flip-Flop1/1 -> Q/1, Scope3/1
  Gain1/1 -> Sum2/2
  Data Type Conversion2/1 -> Scope3/3, S-R Flip-Flop1/1
  Comparator1/1 -> Scope3/2, S-R Flip-Flop1/2
  Sum1/1 -> PID Controller1/1
  Voltage Controller Reference/1 -> Sum1/1
  Pulse Generator1/1 -> Data Type Conversion2/1
  Voltage Sensor Gain/1 -> Sum1/2
  Saturation/1 -> iRef/1, Comparator1/2
  Current Sensor Gain/1 -> Sum2/1
  PID Controller1/1 -> Saturation/1
  In2/1 -> Current Sensor Gain/1
  In1/1 -> Voltage Sensor Gain/1
  Sawtooth Generator/1 -> Gain2/1
  Gain2/1 -> Scope/1, Sum3/1
  Constant/1 -> Sum3/2
  Sum3/1 -> Gain1/1

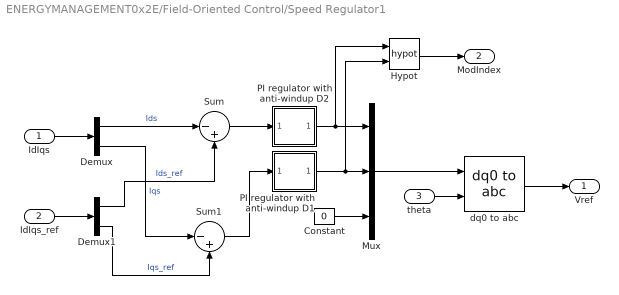
== system ENERGYMANAGEMENT0x2E/Field-Oriented Control/Speed Regulator1 ==
  IdIqs : Inport  PortDimensions=2
  IdIqs_ref : Inport  Port=2  PortDimensions=2
  theta : Inport  Port=3  PortDimensions=1
  Constant : Constant  Value=0
  Demux : Demux  Outputs=2
  Demux1 : Demux  Outputs=2
  Hypot : Math  Operator=hypot
  Mux : Mux  Inputs=3
  PI regulator with anti-windup D1 : Subsystem  DialogController=POWERSYS.PowerSysDialog  mask(Discrete PI Controller){Kp=Kp, Ki=Ki, Par_Limits=[Limits -Limits], Init=0, Ts=Ts}
      mask prompts: Kp "Proportional gain (Kp):"; Ki "Integral gain (Ki):"; Par_Limits "Output limits: [ Upper   Lower ]"; Init "Output initial value:"; Ts "Sample time:"
      mask help: This block implements a discrete PI controller.
      mask init:
      | UpperLimit=Par_Limits(1);
      | LowerLimit=Par_Limits(2);
      | power_initmask();
      mask Help: This block is part of a subset of blocks in the Extras library that does not have documentation associated with it, other than the block mask description.
      mask Display: disp('PI');
  PI regulator with anti-windup D2 : Subsystem  DialogController=POWERSYS.PowerSysDialog  mask(Discrete PI Controller){Kp=Kp, Ki=Ki, Par_Limits=[Limits -Limits], Init=0, Ts=Ts}
      mask prompts: Kp "Proportional gain (Kp):"; Ki "Integral gain (Ki):"; Par_Limits "Output limits: [ Upper   Lower ]"; Init "Output initial value:"; Ts "Sample time:"
      mask help: This block implements a discrete PI controller.
      mask init:
      | UpperLimit=Par_Limits(1);
      | LowerLimit=Par_Limits(2);
      | power_initmask();
      mask Help: This block is part of a subset of blocks in the Extras library that does not have documentation associated with it, other than the block mask description.
      mask Display: disp('PI');
  Sum : Sum  Inputs=|-+
  Sum1 : Sum  Inputs=|-+
  dq0 to abc : spsdq0toabcLib/dq0 to abc  Alignment=90 degrees behind phase A axis
  Vref : Outport
  ModIndex : Outport  Port=2
  wires:
  Hypot/1 -> ModIndex/1
  dq0 to abc/1 -> Vref/1
  Demux1/1 -> Sum/2  "Ids_ref"
  Demux/1 -> Sum/1  "Ids"
  Demux1/2 -> Sum1/2  "Iqs_ref"
  IdIqs_ref/1 -> Demux1/1
  IdIqs/1 -> Demux/1
  PI regulator with anti-windup D2/1(Out) -> Mux/1, Hypot/1
  Sum/1 -> PI regulator with anti-windup D2/1(Error)
  PI regulator with anti-windup D1/1(Out) -> Mux/2, Hypot/2
  Constant/1 -> Mux/3
  Sum1/1 -> PI regulator with anti-windup D1/1(Error)
  Mux/1 -> dq0 to abc/1
  theta/1 -> dq0 to abc/2
  Demux/2 -> Sum1/1  "Iqs"

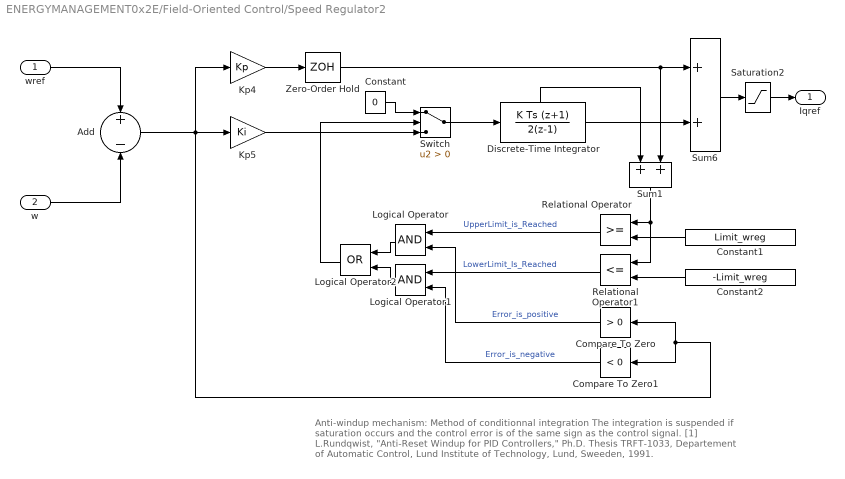
== system ENERGYMANAGEMENT0x2E/Field-Oriented Control/Speed Regulator2 ==
  note: Anti-windup mechanism: Method of conditionnal integration
      |
      | The integration is suspended if saturation occurs and the
      | control error is of the same sign as the control signal.
      |
      | [1] L.Rundqwist, "Anti-Reset Windup for PID Controllers," Ph.D. Thesis TRFT-1033,
      | Departement of Automatic Control, Lund Institute of Technology, Lund, Sweeden, 1991.
  wref : Inport  PortDimensions=1
  w : Inport  Port=2  PortDimensions=1
  Add : Sum  Inputs=+|-
  Compare To Zero : simulink/Logic and Bit Operations/Compare To Zero  relop=>  OutDataTypeStr=uint8  ZeroCross=off
  Compare To Zero1 : simulink/Logic and Bit Operations/Compare To Zero  relop=<  OutDataTypeStr=uint8  ZeroCross=off
  Constant : Constant  Value=0
  Constant1 : Constant  Value=Limit_wreg
  Constant2 : Constant  Value=-Limit_wreg
  Discrete-Time Integrator : DiscreteIntegrator  IntegratorMethod=Integration: Trapezoidal  InitialCondition=Init  SampleTime=Ts  LimitOutput=on  UpperSaturationLimit=Limit_wreg  LowerSaturationLimit=-Limit_wreg  ShowStatePort=on  ICPrevOutput=DiscIntNeverNeededParam  ICPrevScaledInput=DiscIntNeverNeededParam
  Kp4 : Gain  Gain=Kp  SaturateOnIntegerOverflow=on  SampleTime=Ts  OutDataTypeStr=Inherit: Same as input  ParamDataTypeStr=Inherit: Same as input
  Kp5 : Gain  Gain=Ki  SaturateOnIntegerOverflow=on  SampleTime=Ts  OutDataTypeStr=Inherit: Same as input  ParamDataTypeStr=Inherit: Same as input
  Logical Operator : Logic  AllPortsSameDT=off  OutDataTypeStr=boolean
  Logical Operator1 : Logic  AllPortsSameDT=off  OutDataTypeStr=boolean
  Logical Operator2 : Logic  Operator=OR  AllPortsSameDT=off  OutDataTypeStr=boolean
  Relational Operator : RelationalOperator  OutDataTypeStr=boolean  InputSameDT=off
  Relational Operator1 : RelationalOperator  Operator=<=  OutDataTypeStr=boolean  InputSameDT=off
  Saturation2 : Saturate  UpperLimit=Limit_wreg  LowerLimit=-Limit_wreg  SampleTime=Ts
  Sum1 : Sum  InputSameDT=on  SaturateOnIntegerOverflow=on  SampleTime=Ts  OutDataTypeStr=Inherit: Same as first input
  Sum6 : Sum  InputSameDT=on  SaturateOnIntegerOverflow=on  SampleTime=Ts  OutDataTypeStr=Inherit: Same as first input
  Switch : Switch  Criteria=u2 > Threshold  SaturateOnIntegerOverflow=off  InputSameDT=off
  Zero-Order Hold : ZeroOrderHold  SampleTime=Ts
  Iqref : Outport  SampleTime=Ts  InitialOutput=0  VectorParamsAs1DForOutWhenUnconnected=off
  wires:
  Kp5/1 -> Switch/3
  Switch/1 -> Discrete-Time Integrator/1
  Saturation2/1 -> Iqref/1
  Discrete-Time Integrator/1 -> Sum6/2
  Kp4/1 -> Zero-Order Hold/1
  Sum6/1 -> Saturation2/1
  Add/1 -> Compare To Zero/1, Compare To Zero1/1, Kp5/1, Kp4/1
  Compare To Zero1/1 -> Logical Operator1/2  "Error_is_negative"
  Logical Operator1/1 -> Logical Operator2/2
  Logical Operator/1 -> Logical Operator2/1
  Compare To Zero/1 -> Logical Operator/2  "Error_is_positive"
  Constant2/1 -> Relational Operator1/2
  Constant1/1 -> Relational Operator/2
  Relational Operator1/1 -> Logical Operator1/1  "LowerLimit_Is_Reached"
  Relational Operator/1 -> Logical Operator/1  "UpperLimit_is_Reached"
  Logical Operator2/1 -> Switch/2
  Sum1/1 -> Relational Operator/1, Relational Operator1/1
  Discrete-Time Integrator/State -> Sum1/1
  Zero-Order Hold/1 -> Sum6/1, Sum1/2
  Constant/1 -> Switch/1
  wref/1 -> Add/1
  w/1 -> Add/2

== system ENERGYMANAGEMENT0x2E/Fuel Cell Block/Flow rate regulator Air ==
  Iref : Inport
  Fcn1 : Fcn  Expr=60000*8.3145*(273+65)*52*u(1)/(4*96485*(1*101325)*0.4288*.21)
  Fcn2 : Fcn  Expr=50*u(1)>40
  Saturation : Saturate  UpperLimit=inf  LowerLimit=0
  Sum : Sum  Inputs=|++
  flow rate : Outport  VectorParamsAs1DForOutWhenUnconnected=off
  wires:
  Saturation/1 -> flow rate/1
  Sum/1 -> Saturation/1
  Fcn1/1 -> Sum/1
  Iref/1 -> Fcn2/1, Fcn1/1
  Fcn2/1 -> Sum/2

== system ENERGYMANAGEMENT0x2E/Fuel Cell Block/Flow rate regulator H2 ==
  Iref : Inport
  Fcn1 : Fcn  Expr=60000*8.3145*(273+65)*52*u(1)/(2*96485*(1.16*101325)*0.9898*.9995)
  Saturation : Saturate  UpperLimit=24  LowerLimit=0
  flow rate : Outport  VectorParamsAs1DForOutWhenUnconnected=off
  wires:
  Fcn1/1 -> Saturation/1
  Saturation/1 -> flow rate/1
  Iref/1 -> Fcn1/1
